simulink model "task3"  (R2024a)
settings: Solver=VariableStepAuto  StartTime=0.0  StopTime=10.0  RelTol=1e-3
model workspace (MAT data in the model file):
  param_k1 = 0.025
settings Model: Creator=janho  LastModifiedBy=janho

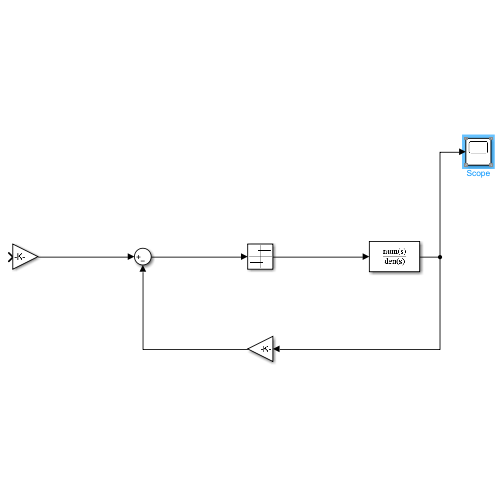
[thumbnail: Simulink's stored preview of the top-level diagram]
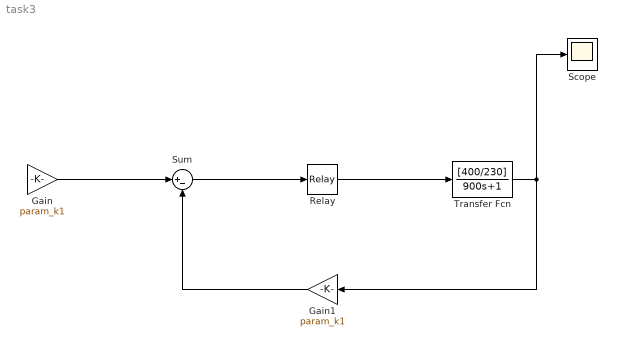
== system task3 ==
  Gain : Gain  Gain=param_k1
  Gain1 : Gain  Gain=param_k1
  Relay : Relay  OnOutputValue=0.2  OffOutputValue=-0.2  OutMax=[230]  ZeroCross=off
  Scope : Scope
  Sum : Sum  Inputs=|+-
  Transfer Fcn : TransferFcn  Numerator=[400/230]  Denominator=[900 1]
  wires:
  Gain1/1 -> Sum/2
  Sum/1 -> Relay/1
  Relay/1 -> Transfer Fcn/1
  Transfer Fcn/1 -> Scope/1, Gain1/1
  Gain/1 -> Sum/1
